simulink model "Pacemaker_A1_01_hardware_hiding"  (R2020a)
settings: Solver=FixedStepAuto  StartTime=0.0  StopTime=10.0  FixedStep=1e-3  RelTol=1e-3  EnableMultiTasking=on
undefined symbols (not defined in the file): D0, D1, D10, D11, D12, D13, D2, D3, D4, D5, D6, D7, D8, D9, PTA0, PTA1, PTA2, PTB23, PTB9, PTC16, PTC17, PTC2, PTC3, PTC4, PTD0, PTD1, PTD2, PTD3
libraries: frdmk64flib x16
settings Model: ExtModeTrigDuration=5  Creator=forre  LastModifiedBy=jeffl
settings OptimizationCC: EnhancedBackFolding=on  PassReuseOutputArgsAs=Individual arguments  ZeroExternalMemoryAtStartup=off  ZeroInternalMemoryAtStartup=off  MaxStackSize=64  OptimizeBlockOrder=speed  DifferentSizesBufferReuse=on  OptimizationCustomize=off  EfficientTunableParamExpr=on
settings DebuggingCC: ParameterTunabilityLossMsg=error
settings HardwareCC: ProdBitPerPointer=32  ProdBitPerSizeT=32  ProdBitPerPtrDiffT=32  ProdLargestAtomicInteger=Long  ProdLargestAtomicFloat=Double  ProdWordSize=32  ProdHWDeviceType=ARM Compatible->ARM Cortex
settings SFSimCC: MATLABDynamicMemAlloc=off
settings RTWCC: SystemTargetFile=ert.tlc  HardwareBoard=NXP FRDM-K64F  TemplateMakefile=ert_default_tmf  Toolchain=GNU Tools for ARM Embedded Processors
settings CodeAppCC: ForceParamTrailComments=on  IgnoreCustomStorageClasses=off  OperatorAnnotations=on  SimulinkDataObjDesc=on  SFDataObjDesc=on  InsertBlockDesc=on

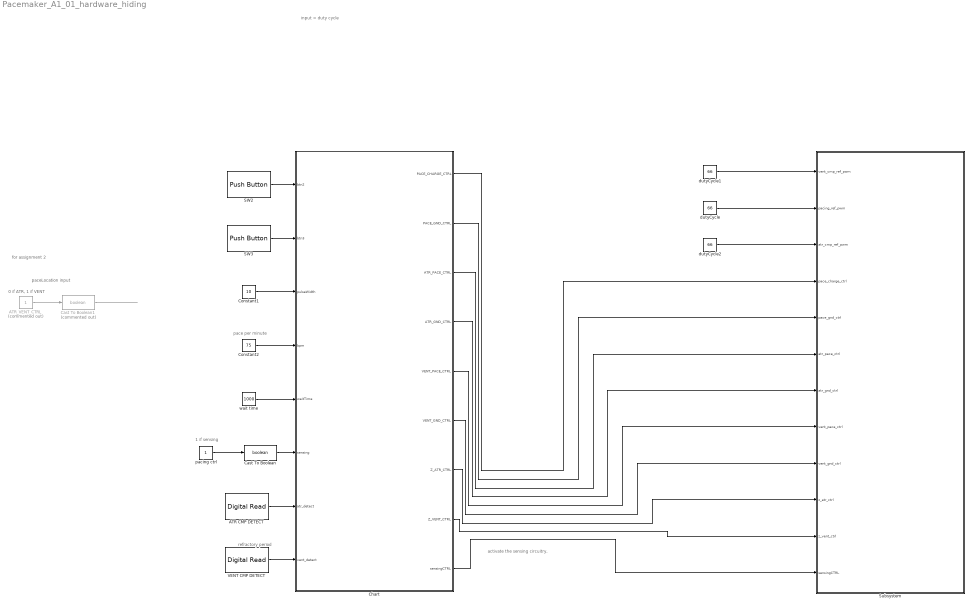
== system Pacemaker_A1_01_hardware_hiding ==
  note: for assignment 2
  note: refractory period
  note: pace per minute
  note: paceLocation input
  note: activate the sensing circuitry.
  note: 0 if ATR, 1 if VENT
  note: input = duty cycle
  note: 1 if sensing
  ATR CMP DETECT : frdmk64flib/Digital Read  Whichpin=PTC16 (D0)  SampleTime=-1
  ATR_VENT_CTRL : Constant  Commented=on
  Cast To Boolean : DataTypeConversion  OutDataTypeStr=boolean
  Cast To Boolean1 : DataTypeConversion  Commented=on  OutDataTypeStr=boolean
  Chart : Stateflow chart  TreatAsAtomicUnit=on
  Constant1 : Constant  Value=10
  Constant2 : Constant  Value=75
  SW2 : frdmk64flib/Push Button  Whichswitch=SW2  SampleTime1=-1
  SW3 : frdmk64flib/Push Button  Whichswitch=SW3  SampleTime1=-1
  Subsystem : Subsystem
  VENT CMP DETECT : frdmk64flib/Digital Read  Whichpin=PTC17 (D1)  SampleTime=-1
  dutyCycle : Constant  Value=66
  dutyCycle1 : Constant  Value=66
  dutyCycle2 : Constant  Value=66
  pacing ctrl : Constant
  wait time : Constant  Value=1000
  wires:
  SW2/1 -> Chart/1(btn2)
  Chart/4(ATR_GND_CTRL) -> Subsystem/7(atr_gnd_ctrl)
  Constant1/1 -> Chart/3(pulseWidth)
  Chart/3(ATR_PACE_CTRL) -> Subsystem/6(atr_pace_ctrl)
  Chart/1(PACE_CHARGE_CTRL) -> Subsystem/4(pace_charge_ctrl)
  Chart/2(PACE_GND_CTRL) -> Subsystem/5(pace_gnd_ctrl)
  Constant2/1 -> Chart/4(bpm)
  Chart/5(VENT_PACE_CTRL) -> Subsystem/8(vent_pace_ctrl)
  Chart/6(VENT_GND_CTRL) -> Subsystem/9(vent_gnd_ctrl)
  Chart/7(Z_ATR_CTRL) -> Subsystem/10(z_atr_ctrl)
  Chart/8(Z_VENT_CTRL) -> Subsystem/11(" z_vent_ctrl")
  ATR_VENT_CTRL/1 -> Cast To Boolean1/1
  pacing ctrl/1 -> Cast To Boolean/1
  ATR CMP DETECT/1 -> Chart/7(atr_detect)
  VENT CMP DETECT/1 -> Chart/8(vent_detect)
  Chart/9(sensingCTRL) -> Subsystem/12(sensingCTRL)
  Cast To Boolean/1 -> Chart/6(sensing)
  Cast To Boolean1/1 -> ?
  SW3/1 -> Chart/2(btn3)
  wait time/1 -> Chart/5(waitTime)
  dutyCycle/1 -> Subsystem/2(pacing_ref_pwm)
  dutyCycle1/1 -> Subsystem/1(vent_cmp_ref_pwm)
  dutyCycle2/1 -> Subsystem/3(atr_cmp_ref_pwm)

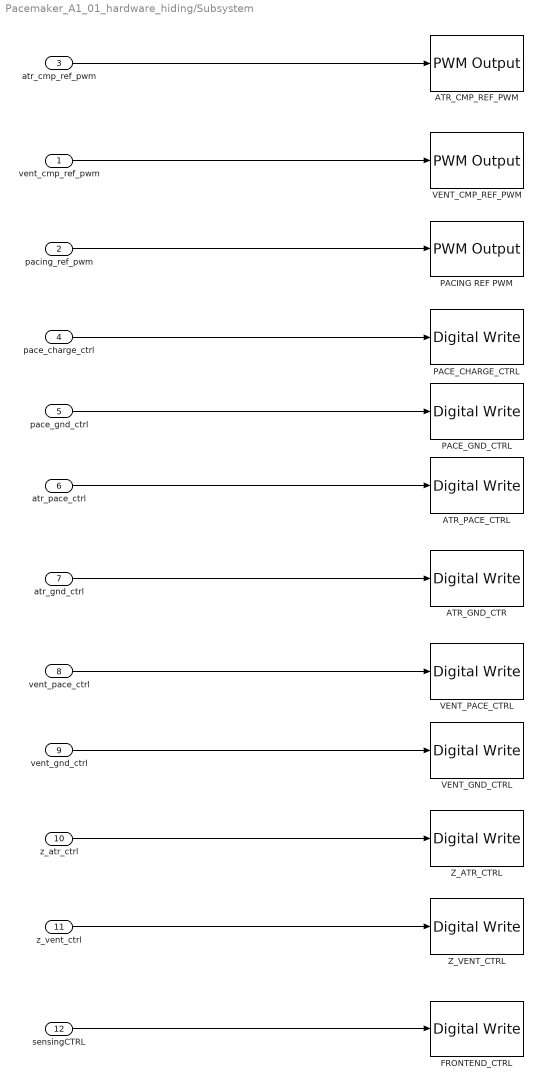
== system Pacemaker_A1_01_hardware_hiding/Subsystem ==
  vent_cmp_ref_pwm : Inport
  pacing_ref_pwm : Inport  Port=2
  atr_cmp_ref_pwm : Inport  Port=3
  pace_charge_ctrl : Inport  Port=4
  pace_gnd_ctrl : Inport  Port=5
  atr_pace_ctrl : Inport  Port=6
  atr_gnd_ctrl : Inport  Port=7
  vent_pace_ctrl : Inport  Port=8
  vent_gnd_ctrl : Inport  Port=9
  z_atr_ctrl : Inport  Port=10
  " z_vent_ctrl" : Inport  Port=11
  sensingCTRL : Inport  Port=12
  ATR_CMP_REF_PWM : frdmk64flib/PWM Output  Whichpin=PTC2 (D6)  InitialFrequency=2000  InitialDutyCycle=50
  ATR_GND_CTR : frdmk64flib/Digital Write  Whichpin=PTD2 (D11)
  ATR_PACE_CTRL : frdmk64flib/Digital Write  Whichpin=PTA0 (D8)
  FRONTEND_CTRL : frdmk64flib/Digital Write  Whichpin=PTD1 (D13)
  PACE_CHARGE_CTRL : frdmk64flib/Digital Write  Whichpin=PTB9 (D2)
  PACE_GND_CTRL : frdmk64flib/Digital Write  Whichpin=PTD0 (D10)
  "PACING REF PWM " : frdmk64flib/PWM Output  Whichpin=PTA2 (D5)  InitialFrequency=2000  InitialDutyCycle=50
  VENT_CMP_REF_PWM : frdmk64flib/PWM Output  Whichpin=PTA1 (D3)  InitialFrequency=2000  InitialDutyCycle=50
  VENT_GND_CTRL : frdmk64flib/Digital Write  Whichpin=PTD3 (D12)
  VENT_PACE_CTRL : frdmk64flib/Digital Write  Whichpin=PTC4 (D9)
  Z_ATR_CTRL : frdmk64flib/Digital Write  Whichpin=PTB23 (D4)
  Z_VENT_CTRL : frdmk64flib/Digital Write  Whichpin=PTC3 (D7)
  wires:
  pace_gnd_ctrl/1 -> PACE_GND_CTRL/1
  atr_pace_ctrl/1 -> ATR_PACE_CTRL/1
  pace_charge_ctrl/1 -> PACE_CHARGE_CTRL/1
  atr_gnd_ctrl/1 -> ATR_GND_CTR/1
  vent_pace_ctrl/1 -> VENT_PACE_CTRL/1
  vent_gnd_ctrl/1 -> VENT_GND_CTRL/1
  z_atr_ctrl/1 -> Z_ATR_CTRL/1
  " z_vent_ctrl"/1 -> Z_VENT_CTRL/1
  sensingCTRL/1 -> FRONTEND_CTRL/1
  pacing_ref_pwm/1 -> "PACING REF PWM "/1
  vent_cmp_ref_pwm/1 -> VENT_CMP_REF_PWM/1
  atr_cmp_ref_pwm/1 -> ATR_CMP_REF_PWM/1

== stateflow chart Pacemaker_A1_01_hardware_hiding/Chart ==
  state SENSING_VENT_TRUE
    entry:
    sensingCTRL = true;
  note: sensing
  state VENT_CHARGING_AND_DISCHARGE
    entry:
    secPerBeat = 60/bpm;
    sensingCTRL = sensing;
    ATR_PACE_CTRL = false;
    VENT_PACE_CTRL = false;
    PACE_CHARGE_CTRL = true;
    PACE_GND_CTRL = true; % 10 in shield expl. doc. diagram
    Z_VENT_CTRL = false;
    Z_ATR_CTRL = false
    VENT_GND_CTRL = true; % 7
    ATR_GND_CTRL = false; % 7
  state VENT_PACING
    entry:
    PACE_GND_CTRL = true; %10
    VENT_PACE_CTRL = true;
    VENT_GND_CTRL = false; %7
    Z_VENT_CTRL = false;
    Z_ATR_CTRL = false;
    ATR_GND_CTRL = false; %7
    ATR_PACE_CTRL = false; % 6
    sensingCTRL = sensing;
  note: VENT PACING
  state changeLocation1
    entry:
    btn2 == false;
  state changeLocation
    entry:
    btn2 == false;
  note: vent
  note: atr
  state ATR_CHARGING_AND_DISCHARGE
    entry:
    secPerBeat = 60/bpm;
    sensingCTRL = sensing;
    ATR_PACE_CTRL = false;
    VENT_PACE_CTRL = false;
    PACE_CHARGE_CTRL = true;
    PACE_GND_CTRL = true; % 10
    Z_VENT_CTRL = false;
    Z_ATR_CTRL = false;
    VENT_GND_CTRL = false; % 7
    ATR_GND_CTRL = true; % 7
  state ATR_PACING
    entry:
    PACE_GND_CTRL = true; %10
    VENT_PACE_CTRL = false;
    VENT_GND_CTRL = false; %7
    Z_VENT_CTRL = false;
    Z_ATR_CTRL = false;
    ATR_GND_CTRL = false; %7
    ATR_PACE_CTRL = true; % 6
    sensingCTRL = sensing;
  note: ATR PACING
  state SENSING_ATR_TRUE
    entry:
    sensingCTRL = true;
  note: sensing
  SENSING_VENT_TRUE -> SENSING_VENT_TRUE [order 2] : [sensingCTRL && (vent_detect || btn3)]
  VENT_PACING -> VENT_CHARGING_AND_DISCHARGE : after(pulseWidth, msec)
  VENT_CHARGING_AND_DISCHARGE -> SENSING_VENT_TRUE [order 3] : [sensingCTRL && (vent_detect || btn3)]
  SENSING_VENT_TRUE -> VENT_CHARGING_AND_DISCHARGE [order 1] : after(waitTime,msec)
  VENT_CHARGING_AND_DISCHARGE -> VENT_PACING [order 1] : after(secPerBeat, sec){PACE_CHARGE_CTRL = false;}
  VENT_CHARGING_AND_DISCHARGE -> changeLocation1 [order 4] : [paceLocation==false]
  changeLocation -> VENT_CHARGING_AND_DISCHARGE : [true]
  VENT_CHARGING_AND_DISCHARGE -> VENT_CHARGING_AND_DISCHARGE [order 2] : [btn2]{paceLocation =false}
  ATR_CHARGING_AND_DISCHARGE -> VENT_CHARGING_AND_DISCHARGE [commented out] : [paceLocation==true]
  VENT_CHARGING_AND_DISCHARGE -> ATR_CHARGING_AND_DISCHARGE [commented out] : [paceLocation==false]
  changeLocation1 -> ATR_CHARGING_AND_DISCHARGE : [true]
  ATR_CHARGING_AND_DISCHARGE -> changeLocation [order 4] : [paceLocation==true]
  (default) -> ATR_CHARGING_AND_DISCHARGE
  ATR_CHARGING_AND_DISCHARGE -> ATR_PACING [order 1] : after(secPerBeat, sec){PACE_CHARGE_CTRL = false;}
  ATR_CHARGING_AND_DISCHARGE -> ATR_CHARGING_AND_DISCHARGE [order 2] : [btn2]{paceLocation = true}
  ATR_CHARGING_AND_DISCHARGE -> SENSING_ATR_TRUE [order 3] : [sensingCTRL && (atr_detect || btn3)]
  SENSING_ATR_TRUE -> ATR_CHARGING_AND_DISCHARGE [order 1] : after(waitTime,msec)
  ATR_PACING -> ATR_CHARGING_AND_DISCHARGE : after(pulseWidth, msec)
  SENSING_ATR_TRUE -> SENSING_ATR_TRUE [order 2] : [sensingCTRL && (atr_detect || btn3)]
  data: PACE_CHARGE_CTRL output boolean; PACE_GND_CTRL output boolean; btn2 input boolean; btn3 input boolean; ATR_PACE_CTRL output boolean; ATR_GND_CTRL output boolean; pulseWidth input double; bpm input double; waitTime input double; secPerBeat local double; VENT_PACE_CTRL output boolean; VENT_GND_CTRL output boolean; Z_ATR_CTRL output boolean; Z_VENT_CTRL output boolean; sensing input boolean; atr_detect input boolean; vent_detect input boolean; sensingCTRL output boolean; paceLocation local boolean
  data atr_detect settings: description=|
      | 0 = pace atrium
      | 1 = pace ventricle
  data vent_detect settings: description=|
      | 0 = pace atrium
      | 1 = pace ventricle
  data paceLocation settings: description=|
      | 0 = pace atrium
      | 1 = pace ventricle
